simulink model "PMSM_FOC_demo"  (R2016a)
settings: Solver=ode3  StartTime=0.0  StopTime=0.4  FixedStep=ts  RelTol=1e-3
InitFcn:
  | para_init;
values from neighbouring files (symbols this model uses):
  J = 0.15    [para_init.m]
  MotOpMod = 2    [para_init.m]
  n_max = 6000    [para_init.m]
  nMotOpSpdMod = 1000*2*pi/60    (= 104.71975512)    [para_init.m]
  pp = 6    [para_init.m]
  r_dq = tan(theta_mtpa)    [para_init.m]
  ts_cc = 1/f_cc    (= 0.0001)    [para_init.m]
  U_bat = 200    [para_init.m]
undefined symbols (not defined in the file or in its folder): sigbuilder_block
undefined symbols (not defined in the file): f_cc, i_max, i_min, Kc_id, Kc_iq, Kc_n, Ki_id, Ki_iq, Ki_n, Kp_id, Kp_iq, Kp_n, Lamda_pm, lpa_cc, lpb_cc, Ls_d, Ls_q, rs, Te_max, Te_min, theta0, ts
libraries: simulink x2, simulink_extras x1
(part 1 of 2)
settings Model: Creator=Xinmei  LastModifiedBy=xinmei
settings DataIOCC: LimitDataPoints=on  SaveFormat=Array  SignalLoggingSaveFormat=ModelDataLogs
settings OptimizationCC: ExpressionDepthLimit=2147483647  EfficientMapNaN2IntZero=off
settings DebuggingCC: UnderspecifiedInitializationDetection=Classic  MergeDetectMultiDrivingBlocksExec=none  SolverPrmCheckMsg=warning  InheritedTsInSrcMsg=none  FcnCallInpInsideContextMsg=UseLocalSettings  StateNameClashWarn=warning
settings HardwareCC: ProdBitPerPointer=32  ProdLargestAtomicFloat=None  ProdIntDivRoundTo=Undefined  ProdEndianess=Unspecified  ProdWordSize=32  ProdHWDeviceType=32-bit Generic  TargetBitPerPointer=64  TargetLongLongMode=on  TargetIntDivRoundTo=Zero  TargetEndianess=LittleEndian  TargetWordSize=64  TargetHWDeviceType=MATLAB Host  ProdEqTarget=off
settings ModelReferenceCC: PropagateSignalLabelsOutOfModel=off
settings CodeAppCC: MaxIdLength=128
settings GRTTargetCC: CombineOutputUpdateFcns=off  GRTInterface=on
settings ConfigComp: CovModelRefEnable=Off

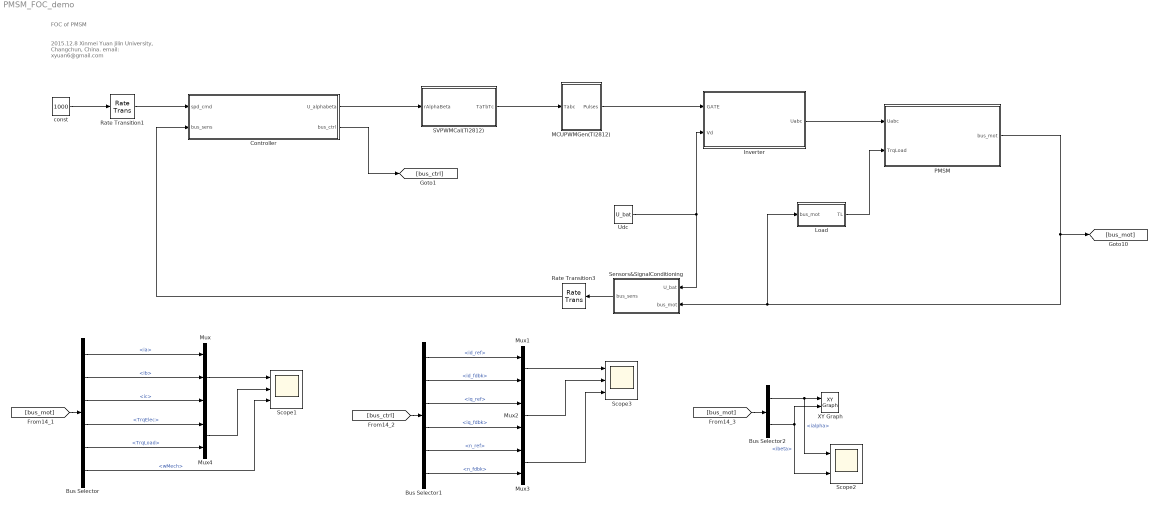
== system PMSM_FOC_demo ==
  note: 2015.12.8 Xinmei Yuan
      | Jilin University, Changchun, China.
      | email: xyuan6@gmail.com
  note: FOC of PMSM
  Bus Selector : BusSelector  OutputSignals=ia,ib,ic,TrqElec,TrqLoad,wMech
  Bus Selector1 : BusSelector  OutputSignals=id_ref,id_fdbk,iq_ref,iq_fdbk,n_ref,n_fdbk
  Bus Selector2 : BusSelector  OutputSignals=ialpha,ibeta
  Controller : Subsystem
  Inverter : Subsystem
      mask Display:
      | %image (imread('IGBT.jpg'))
      | port_label('input',1,'Gate'  )
      | port_label('input',2,'Udc'  )
      | port_label('output',1,'Uabc')
  Load : Subsystem
  MCUPWMGen(TI2812) : Subsystem  mask{fpwm=f_cc, nbit=16, Pulselim=0}
      mask prompts: fpwm "Chopping frequency(Hz)"; nbit "MCU PWM bits (ie: 16bits)"; Pulselim "PWM Pulse filtered"
  Mux : Mux  Inputs=3
  Mux{1..4} (4 alike) : Mux  Inputs=2
  PMSM : Subsystem  mask{r=rs, Ld=Ls_d, Lq=Ls_q, lamdaPM=Lamda_pm, J=J, p=pp, Thetam_init=theta0}
      mask prompts: r "Resistance (Ohm)"; Ld "Inductance Ld (H)"; Lq "Inductance Lq (H)"; lamdaPM "Flux induced by magnets (Wb)"; J "Inertia (kg*m^2)"; p "Pairs of poles"; Thetam_init "Rotor Initial Angle (rad)"
      mask Display:
      | %image (imread('Motor.jpg'))
      | port_label('input',1,'Uabc'  )
      | port_label('input',2,'T_L'  )
      | port_label('output',1,'bus_mot')
  Rate Transition1 : RateTransition  Integrity=off  OutPortSampleTime=ts_cc
  Rate Transition3 : RateTransition  Integrity=off  OutPortSampleTime=ts_cc
  SVPWMCal(TI2812) : Subsystem  mask{fpwm=f_cc}
      mask prompts: fpwm "Chopping frequency (Hz):"
      mask Display:
      | %image (imread('SVPWM.jpg'))
      | port_label('input',1,'rAlphaBeta'  )
      | port_label('output',1,'Tabc')
  Scope1 : Scope  NumInputPorts=3
  Scope2 : Scope  NumInputPorts=2
  Scope3 : Scope  NumInputPorts=3
  Sensors&SignalConditioning : Subsystem
  Udc : Constant  Value=U_bat  SampleTime=0
  XY Graph : simulink/Sinks/XY Graph  xmin=-150  xmax=150  ymin=-150  ymax=150  st=-1
  const : Constant  Value=1000  SampleTime=0
  wires:
  MCUPWMGen(TI2812)/1(Pulses) -> Inverter/1(GATE)
  Inverter/1(Uabc) -> PMSM/1(Uabc)
  SVPWMCal(TI2812)/1(TaTbTc) -> MCUPWMGen(TI2812)/1(Tabc)
  Udc/1 -> Sensors&SignalConditioning/1(U_bat), Inverter/2(Vd)
  PMSM/1(bus_mot) -> Load/1(bus_mot), Sensors&SignalConditioning/2(bus_mot), [bus_mot]
  [bus_mot] -> Bus Selector/1
  Bus Selector/3 -> Mux/3  "<ic>"
  Bus Selector/2 -> Mux/2  "<ib>"
  Bus Selector/1 -> Mux/1  "<ia>"
  Mux/1 -> Scope1/1
  Bus Selector/6 -> Scope1/3  "<wMech>"
  Load/1(TL) -> PMSM/2(TrqLoad)
  Sensors&SignalConditioning/1(bus_sens) -> Rate Transition3/1
  Rate Transition3/1 -> Controller/2(bus_sens)
  Controller/1(U_alphabeta) -> SVPWMCal(TI2812)/1(rAlphaBeta)
  const/1 -> Rate Transition1/1
  Rate Transition1/1 -> Controller/1(spd_cmd)
  [bus_ctrl] -> Bus Selector1/1
  Controller/2(bus_ctrl) -> [bus_ctrl]
  Bus Selector1/1 -> Mux1/1  "<id_ref>"
  Bus Selector1/2 -> Mux1/2  "<id_fdbk>"
  Bus Selector1/3 -> Mux2/1  "<iq_ref>"
  Bus Selector1/4 -> Mux2/2  "<iq_fdbk>"
  Mux1/1 -> Scope3/1
  Mux2/1 -> Scope3/2
  Bus Selector1/5 -> Mux3/1  "<n_ref>"
  Bus Selector1/6 -> Mux3/2  "<n_fdbk>"
  Mux3/1 -> Scope3/3
  Bus Selector/4 -> Mux4/1  "<TrqElec>"
  Bus Selector/5 -> Mux4/2  "<TrqLoad>"
  Mux4/1 -> Scope1/2
  [bus_mot] -> Bus Selector2/1
  Bus Selector2/1 -> Scope2/1, XY Graph/1  "<ialpha>"
  Bus Selector2/2 -> XY Graph/2, Scope2/2  "<ibeta>"

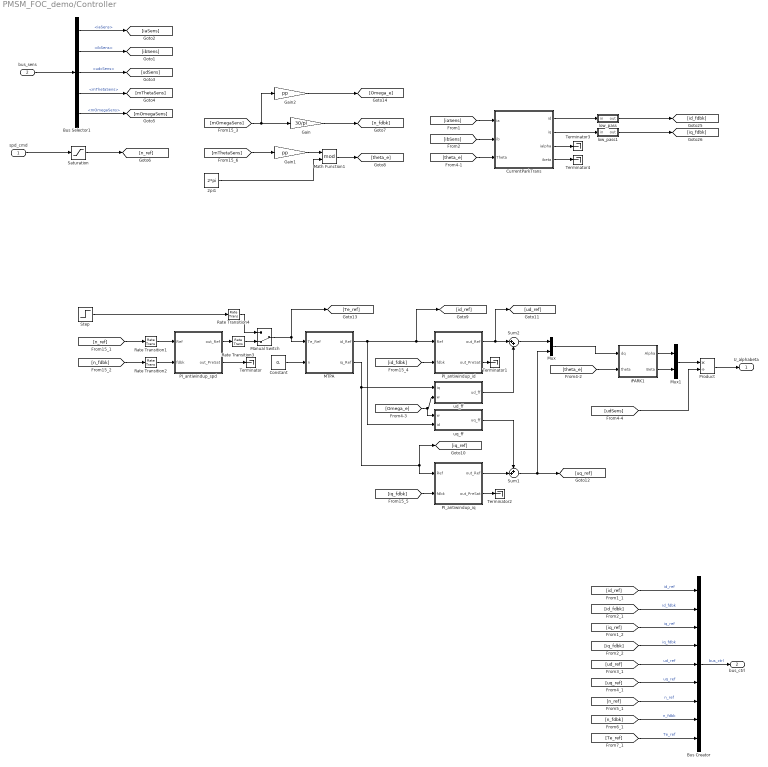
== system PMSM_FOC_demo/Controller ==
  spd_cmd : Inport
  bus_sens : Inport  Port=2
  2pi1 : Constant  Value=2*pi  SampleTime=ts_cc
  Bus Creator : BusCreator  Inputs=9
  Bus Selector1 : BusSelector  OutputSignals=iaSens,ibSens,udcSens,mThetaSens,mOmegaSens
  Constant : Constant  Value=0.  SampleTime=0
  CurrentParkTrans : Subsystem
  Gain : Gain  Gain=30/pi  SaturateOnIntegerOverflow=on  OutDataTypeStr=Inherit: Same as input  ParamDataTypeStr=Inherit: Same as input
  Gain1 : Gain  Gain=pp  SaturateOnIntegerOverflow=on  OutDataTypeStr=Inherit: Same as input  ParamDataTypeStr=Inherit: Same as input
  Gain2 : Gain  Gain=pp  SaturateOnIntegerOverflow=on  OutDataTypeStr=Inherit: Same as input  ParamDataTypeStr=Inherit: Same as input
  MTPA : Subsystem
  Manual Switch : ManualSwitch  CurrentSetting=0
  Math Function1 : Math  Operator=mod  SaturateOnIntegerOverflow=on
  Mux : Mux  Inputs=2
  Mux1 : Mux  Inputs=2
  PI_antiwindup_id : Subsystem  mask(PI Controller){P=Kp_id, I=Ki_id, sat=[i_min,i_max], Kc=Kc_id}
      mask prompts: P "Proportional:"; I "Integral"; sat "Minimum and maximum outputs:"
      mask init:
      | min=sat(1);max=sat(2);
  PI_antiwindup_iq : Subsystem  mask(PI Controller){P=Kp_iq, I=Ki_iq, sat=[i_min,i_max], Kc=Kc_iq}
      mask prompts: P "Proportional:"; I "Integral"; sat "Minimum and maximum outputs:"
      mask init:
      | min=sat(1);max=sat(2);
  PI_antiwindup_spd : Subsystem  mask(PI Controller){P=Kp_n, I=Ki_n, sat=[Te_min,Te_max], Kc=Kc_n}
      mask prompts: P "Proportional:"; I "Integral"; sat "Minimum and maximum outputs:"
      mask init:
      | min=sat(1);max=sat(2);
  Product : Product  Inputs=*/  SaturateOnIntegerOverflow=on  OutDataTypeStr=Inherit: Same as first input
  Rate Transition1 : RateTransition  Integrity=off  OutPortSampleTime=ts_sc
  Rate Transition2 : RateTransition  Integrity=off  OutPortSampleTime=ts_sc
  Rate Transition3 : RateTransition  Integrity=off  OutPortSampleTime=ts_cc
  Rate Transition4 : RateTransition  Integrity=off  OutPortSampleTime=ts_cc
  Saturation : Saturate  UpperLimit=n_max  LowerLimit=-n_max
  Step : Step  Time=0.5  After=10  SampleTime=ts_cc
  Sum1 : Sum  Inputs=++|
  Sum2 : Sum  Inputs=|++
  Terminator{,1..4} (5 alike) : Terminator
  iPARK1 : Subsystem
  low_pass : Subsystem  mask{a=lpa_cc, b=lpb_cc}
  low_pass1 : Subsystem  mask{a=lpa_cc, b=lpb_cc}
  ud_ff : Subsystem  mask{Lq=Ls_q}
  uq_ff : Subsystem  mask{Ld=Ls_d, lamdaPM=Lamda_pm}
  U_alphabeta : Outport
  bus_ctrl : Outport  Port=2
  wires:
  bus_sens/1 -> Bus Selector1/1
  Bus Selector1/1 -> [iaSens]  "<iaSens>"
  Bus Selector1/2 -> [ibSens]  "<ibSens>"
  Bus Selector1/3 -> [udSens]  "<udcSens>"
  Bus Selector1/4 -> [mThetaSens]  "<mThetaSens>"
  Bus Selector1/5 -> [mOmegaSens]  "<mOmegaSens>"
  [mOmegaSens] -> Gain2/1, Gain/1
  Gain/1 -> [n_fdbk]
  Saturation/1 -> [n_ref]
  [n_ref] -> Rate Transition1/1
  [n_fdbk] -> Rate Transition2/1
  PI_antiwindup_spd/2(out_PreSat) -> Terminator/1
  Constant/1 -> MTPA/2(n)
  Step/1 -> Rate Transition4/1
  PI_antiwindup_spd/1(out_Ref) -> Rate Transition3/1
  [id_fdbk] -> PI_antiwindup_id/2(fdbk)
  MTPA/1(id_Ref) -> uq_ff/2(id), [id_ref], PI_antiwindup_id/1(Ref)
  [iq_fdbk] -> PI_antiwindup_iq/2(fdbk)
  MTPA/2(iq_Ref) -> ud_ff/1(iq), PI_antiwindup_iq/1(Ref), [iq_ref]
  PI_antiwindup_id/2(out_PreSat) -> Terminator1/1
  PI_antiwindup_iq/2(out_PreSat) -> Terminator2/1
  Mux/1 -> iPARK1/1(dq)
  [theta_e] -> CurrentParkTrans/3(Theta)
  CurrentParkTrans/1(id) -> low_pass/1(in)
  CurrentParkTrans/2(iq) -> low_pass1/1(in)
  [iaSens] -> CurrentParkTrans/1(ia)
  [ibSens] -> CurrentParkTrans/2(ib)
  [mThetaSens] -> Gain1/1
  Gain1/1 -> Math Function1/1
  Math Function1/1 -> [theta_e]
  CurrentParkTrans/3(ialpha) -> Terminator3/1
  CurrentParkTrans/4(ibeta) -> Terminator4/1
  [theta_e] -> iPARK1/2(theta)
  2pi1/1 -> Math Function1/2
  Bus Creator/1 -> bus_ctrl/1  "bus_ctrl"
  [id_ref] -> Bus Creator/1  "id_ref"
  [id_fdbk] -> Bus Creator/2  "id_fdbk"
  [iq_ref] -> Bus Creator/3  "iq_ref"
  [iq_fdbk] -> Bus Creator/4  "iq_fdbk"
  Mux1/1 -> Product/1
  iPARK1/1(Alpha) -> Mux1/1
  iPARK1/2(Beta) -> Mux1/2
  [ud_ref] -> Bus Creator/5  "ud_ref"
  [uq_ref] -> Bus Creator/6  "uq_ref"
  low_pass/1(out) -> [id_fdbk]
  low_pass1/1(out) -> [iq_fdbk]
  [Omega_e] -> uq_ff/1(w), ud_ff/2(w)
  PI_antiwindup_id/1(out_Ref) -> Sum2/1, [ud_ref]
  uq_ff/1(uq_ff) -> Sum1/1
  PI_antiwindup_iq/1(out_Ref) -> Sum1/2
  ud_ff/1(ud_ff) -> Sum2/2
  Product/1 -> U_alphabeta/1
  [udSens] -> Product/2
  Sum2/1 -> Mux/1
  Sum1/1 -> Mux/2, [uq_ref]
  spd_cmd/1 -> Saturation/1
  Rate Transition2/1 -> PI_antiwindup_spd/2(fdbk)
  Manual Switch/1 -> MTPA/1(Te_Ref), [Te_ref]
  Rate Transition3/1 -> Manual Switch/2
  [n_ref] -> Bus Creator/7  "n_ref"
  [n_fdbk] -> Bus Creator/8  "n_fdbk"
  [Te_ref] -> Bus Creator/9  "Te_ref"
  Rate Transition1/1 -> PI_antiwindup_spd/1(Ref)
  Rate Transition4/1 -> Manual Switch/1
  Gain2/1 -> [Omega_e]

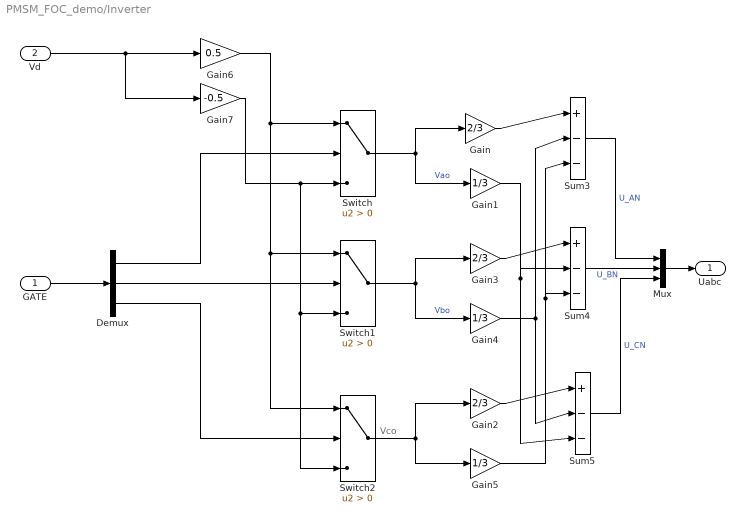
== system PMSM_FOC_demo/Inverter ==
  note: Vco
  GATE : Inport
  Vd : Inport  Port=2
  Demux : Demux  Outputs=3
  Gain : Gain  Gain=2/3  SaturateOnIntegerOverflow=on  OutDataTypeStr=Inherit: Same as input  ParamDataTypeStr=Inherit: Same as input
  Gain1 : Gain  Gain=1/3  SaturateOnIntegerOverflow=on  OutDataTypeStr=Inherit: Same as input  ParamDataTypeStr=Inherit: Same as input
  Gain2 : Gain  Gain=2/3  SaturateOnIntegerOverflow=on  OutDataTypeStr=Inherit: Same as input  ParamDataTypeStr=Inherit: Same as input
  Gain3 : Gain  Gain=2/3  SaturateOnIntegerOverflow=on  OutDataTypeStr=Inherit: Same as input  ParamDataTypeStr=Inherit: Same as input
  Gain4 : Gain  Gain=1/3  SaturateOnIntegerOverflow=on  OutDataTypeStr=Inherit: Same as input  ParamDataTypeStr=Inherit: Same as input
  Gain5 : Gain  Gain=1/3  SaturateOnIntegerOverflow=on  OutDataTypeStr=Inherit: Same as input  ParamDataTypeStr=Inherit: Same as input
  Gain6 : Gain  Gain=0.5  SaturateOnIntegerOverflow=on  OutDataTypeStr=Inherit: Same as input  ParamDataTypeStr=Inherit: Same as input
  Gain7 : Gain  Gain=-0.5  SaturateOnIntegerOverflow=on  OutDataTypeStr=Inherit: Same as input  ParamDataTypeStr=Inherit: Same as input
  Mux : Mux  Inputs=3
  Sum3 : Sum  Inputs=|+--  SaturateOnIntegerOverflow=on
  Sum4 : Sum  Inputs=|+--  SaturateOnIntegerOverflow=on
  Sum5 : Sum  Inputs=|+--  SaturateOnIntegerOverflow=on
  Switch : Switch  Criteria=u2 > Threshold  SaturateOnIntegerOverflow=on
  Switch1 : Switch  Criteria=u2 > Threshold  SaturateOnIntegerOverflow=on
  Switch2 : Switch  Criteria=u2 > Threshold  SaturateOnIntegerOverflow=on
  Uabc : Outport
  wires:
  GATE/1 -> Demux/1
  Demux/3 -> Switch2/2
  Demux/2 -> Switch1/2
  Demux/1 -> Switch/2
  Mux/1 -> Uabc/1
  Sum5/1 -> Mux/3  "U_CN"
  Sum4/1 -> Mux/2  "U_BN"
  Sum3/1 -> Mux/1  "U_AN"
  Vd/1 -> Gain7/1, Gain6/1
  Gain2/1 -> Sum5/1
  Gain1/1 -> Sum5/3, Sum4/2
  Gain3/1 -> Sum4/1
  Gain5/1 -> Sum4/3, Sum3/3
  Gain4/1 -> Sum5/2, Sum3/2
  Gain/1 -> Sum3/1
  Switch2/1 -> Gain5/1, Gain2/1
  Switch1/1 -> Gain4/1, Gain3/1  "Vbo"
  Switch/1 -> Gain1/1, Gain/1  "Vao"
  Gain7/1 -> Switch1/3, Switch2/3, Switch/3
  Gain6/1 -> Switch1/1, Switch2/1, Switch/1

== system PMSM_FOC_demo/Load ==
  bus_mot : Inport
  Bus Selector : BusSelector  OutputSignals=wMech
  Constant : Constant  Value=0  SampleTime=0
  Gain : Gain  Gain=30/pi  SaturateOnIntegerOverflow=on  OutDataTypeStr=Inherit: Same as input  ParamDataTypeStr=Inherit: Same as input
  Gain1 : Gain  Gain=0.01  SaturateOnIntegerOverflow=on  OutDataTypeStr=Inherit: Same as input  ParamDataTypeStr=Inherit: Same as input
  Manual Switch : ManualSwitch  CurrentSetting=0
  Signal Builder : Subsystem  Tag=STV Subsys  LoadFcn=sigbuilder_block('load');  StartFcn=sigbuilder_block('start');  StopFcn=sigbuilder_block('stop');  ClipboardFcn=sigbuilder_block('clipboard');  mask(Sigbuilder block){}
      mask help: Simulink:masks:SigbuilderBlock_MD
      mask init:
      | if ~strcmp(get_param(bdroot(gcbh),'SimulationStatus'),'stopped') tuvar = sigbuilder_block('maskInit'); end
      settings: CopyFcn=sigbuilder_block('copy');  DeleteFcn=sigbuilder_block('delete');  ModelCloseFcn=sigbuilder_block('modelClose');  PreSaveFcn=sigbuilder_block('preSave');  PauseFcn=sigbuilder_block('pause');  ContinueFcn=sigbuilder_block('continue');  NameChangeFcn=sigbuilder_block('namechange');  OpenFcn=sigbuilder_block('open',[437.25 199.5 550.5 399.75 ]);  CloseFcn=sigbuilder_block('close');
      mask Display: plot(0, 0, 100, 100,[2, 2, 32, 32, 2], [68, 8, 8, 68, 68],[32, 2], [38, 38], [32, 19, 2],[53, 60, 44], [32, 17, 17, 2],[16, 16, 31, 31]);txt = getActiveGroup(gcbh);text(2, 100, txt,'verticalAlignment', 'top');
  Sum : Sum  Inputs=|++
  TL : Outport
  wires:
  Bus Selector/1 -> [wMech]  "<wMech>"
  bus_mot/1 -> Bus Selector/1
  [wMech] -> Gain/1
  Gain/1 -> Gain1/1
  Gain1/1 -> Sum/1
  Sum/1 -> TL/1
  Constant/1 -> Manual Switch/1
  Manual Switch/1 -> Sum/2
  Signal Builder/1(Imported_Signal 1) -> Manual Switch/2

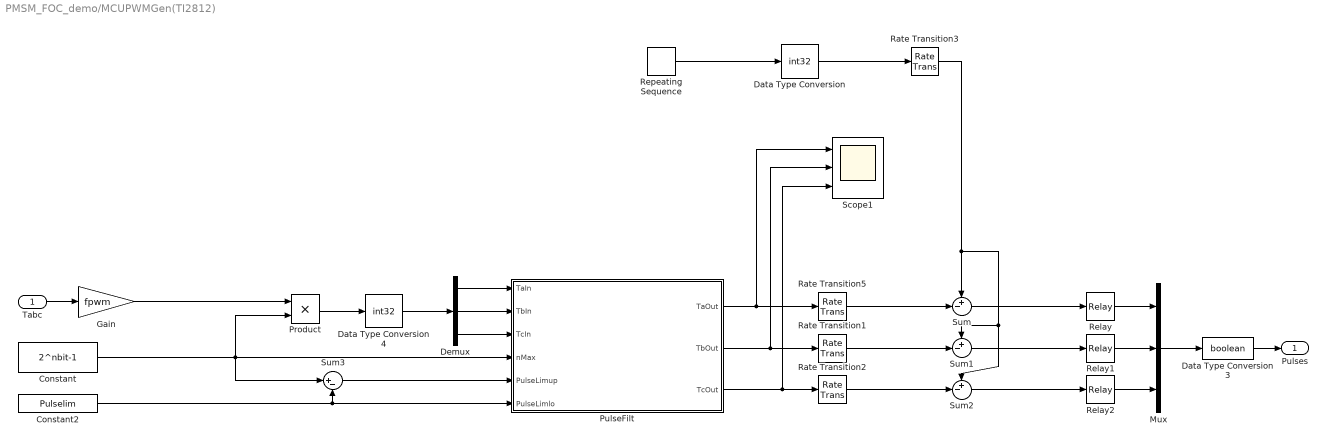
== system PMSM_FOC_demo/MCUPWMGen(TI2812) ==
  Tabc : Inport
  Constant : Constant  Value=2^nbit-1
  Constant2 : Constant  Value=Pulselim
  Data Type Conversion : DataTypeConversion  OutDataTypeStr=int32
  Data Type Conversion3 : DataTypeConversion  OutDataTypeStr=boolean
  Data Type Conversion4 : DataTypeConversion  OutDataTypeStr=int32
  Demux : Demux  Outputs=3
  Gain : Gain  Gain=fpwm
  Mux : Mux  Inputs=3
  Product : Product  RndMeth=Zero
  PulseFilt : Stateflow chart  TreatAsAtomicUnit=on
  Rate Transition{1..3,5} (4 alike) : RateTransition  Integrity=off  OutPortSampleTime=0
  Relay : Relay  OnSwitchValue=1  OffSwitchValue=-1
  Relay1 : Relay  OnSwitchValue=1  OffSwitchValue=-1
  Relay2 : Relay  OnSwitchValue=1  OffSwitchValue=-1
  Repeating Sequence : simulink/Sources/Repeating Sequence  rep_seq_t=[0 1/2/fpwm 1/fpwm]  rep_seq_y=[0 2^nbit-1 0]
  Scope1 : Scope  NumInputPorts=3
  Sum : Sum  Inputs=+-|
  Sum1 : Sum  Inputs=+-|
  Sum2 : Sum  Inputs=+-|
  Sum3 : Sum  Inputs=|+-
  Pulses : Outport
  wires:
  Data Type Conversion3/1 -> Pulses/1
  Repeating Sequence/1 -> Data Type Conversion/1
  Mux/1 -> Data Type Conversion3/1
  Tabc/1 -> Gain/1
  Relay2/1 -> Mux/3
  Relay1/1 -> Mux/2
  Relay/1 -> Mux/1
  Sum2/1 -> Relay2/1
  Sum1/1 -> Relay1/1
  Sum/1 -> Relay/1
  Data Type Conversion/1 -> Rate Transition3/1
  PulseFilt/1(TaOut) -> Scope1/1, Rate Transition5/1
  PulseFilt/2(TbOut) -> Scope1/2, Rate Transition1/1
  PulseFilt/3(TcOut) -> Scope1/3, Rate Transition2/1
  Data Type Conversion4/1 -> Demux/1
  Product/1 -> Data Type Conversion4/1
  Gain/1 -> Product/1
  Constant/1 -> Product/2, PulseFilt/4(nMax), Sum3/1
  Demux/1 -> PulseFilt/1(TaIn)
  Demux/2 -> PulseFilt/2(TbIn)
  Demux/3 -> PulseFilt/3(TcIn)
  Sum3/1 -> PulseFilt/5(PulseLimup)
  Constant2/1 -> PulseFilt/6(PulseLimlo), Sum3/2
  Rate Transition5/1 -> Sum/2
  Rate Transition1/1 -> Sum1/2
  Rate Transition2/1 -> Sum2/2
  Rate Transition3/1 -> Sum/1, Sum2/1, Sum1/1

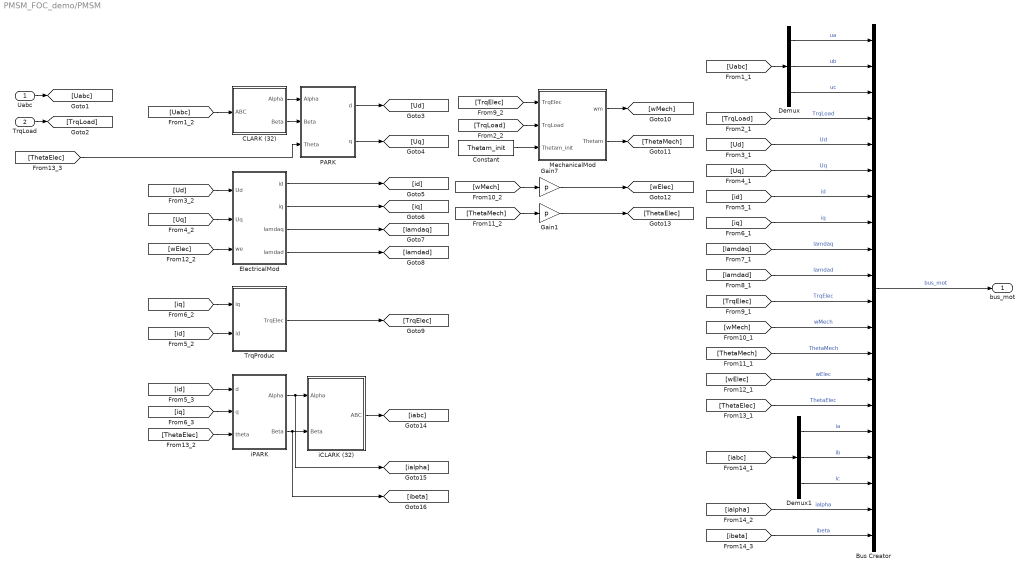
== system PMSM_FOC_demo/PMSM ==
  Uabc : Inport
  TrqLoad : Inport  Port=2
  Bus Creator : BusCreator  Inputs=20
  CLARK (32) : Subsystem
  Constant : Constant  Value=Thetam_init  SampleTime=[0, 0]
  Demux : Demux  Outputs=3
  Demux1 : Demux  Outputs=3
  ElectricalMod : Subsystem  mask{r=r, Ld=Ld, Lq=Lq, lamdaPM=lamdaPM}
      mask prompts: r "Stator resistance"; Ld "d axis inductance"; Lq "q axis inductance"; lamdaPM "Flux induced by magnets"
  Gain1 : Gain  Gain=p  SaturateOnIntegerOverflow=on  OutDataTypeStr=Inherit: Same as input  ParamDataTypeStr=Inherit: Same as input
  Gain7 : Gain  Gain=p  SaturateOnIntegerOverflow=on  OutDataTypeStr=Inherit: Same as input  ParamDataTypeStr=Inherit: Same as input
  MechanicalMod : Subsystem  mask{J=J}
      mask prompts: J "Intertia (kg*m^2)"
  PARK : Subsystem
  TrqProduc : Subsystem  mask{Ld=Ld, Lq=Lq, lamdaPM=lamdaPM, p=p}
      mask prompts: Ld "d Axis inductance"; Lq "q Axis inductance"; lamdaPM "Flux induced by magnets"; p "Pairs of poles"
  iCLARK (32) : Subsystem
  iPARK : Subsystem
  bus_mot : Outport
  wires:
  Bus Creator/1 -> bus_mot/1  "bus_mot"
  Demux1/3 -> Bus Creator/18  "ic"
  Demux1/2 -> Bus Creator/17  "ib"
  Demux1/1 -> Bus Creator/16  "ia"
  [ThetaElec] -> Bus Creator/15  "ThetaElec"
  [wElec] -> Bus Creator/14  "wElec"
  [ThetaMech] -> Bus Creator/13  "ThetaMech"
  [wMech] -> Bus Creator/12  "wMech"
  [TrqElec] -> Bus Creator/11  "TrqElec"
  [lamdad] -> Bus Creator/10  "lamdad"
  [lamdaq] -> Bus Creator/9  "lamdaq"
  [iq] -> Bus Creator/8  "iq"
  [id] -> Bus Creator/7  "id"
  [Uq] -> Bus Creator/6  "Uq"
  [Ud] -> Bus Creator/5  "Ud"
  [TrqLoad] -> Bus Creator/4  "TrqLoad"
  Demux/3 -> Bus Creator/3  "uc"
  Demux/2 -> Bus Creator/2  "ub"
  Demux/1 -> Bus Creator/1  "ua"
  [iabc] -> Demux1/1
  [Uabc] -> Demux/1
  [ThetaElec] -> iPARK/3(theta)
  [id] -> iPARK/1(d)
  iCLARK (32)/1(ABC) -> [iabc]
  [wElec] -> ElectricalMod/3(we)
  [ThetaMech] -> Gain1/1
  Gain7/1 -> [wElec]
  [wMech] -> Gain7/1
  MechanicalMod/2(Thetam) -> [ThetaMech]
  MechanicalMod/1(wm) -> [wMech]
  ElectricalMod/4(lamdad) -> [lamdad]
  ElectricalMod/3(lamdaq) -> [lamdaq]
  Constant/1 -> MechanicalMod/3(Thetam_init)
  [TrqLoad] -> MechanicalMod/2(TrqLoad)
  [TrqElec] -> MechanicalMod/1(TrqElec)
  TrqProduc/1(TrqElec) -> [TrqElec]
  ElectricalMod/2(iq) -> [iq]
  ElectricalMod/1(id) -> [id]
  [Uq] -> ElectricalMod/2(Uq)
  [Ud] -> ElectricalMod/1(Ud)
  PARK/2(q) -> [Uq]
  PARK/1(d) -> [Ud]
  TrqLoad/1 -> [TrqLoad]
  [Uabc] -> CLARK (32)/1(ABC)
  Uabc/1 -> [Uabc]
  [iq] -> TrqProduc/1(iq)
  [id] -> TrqProduc/2(id)
  CLARK (32)/1(Alpha) -> PARK/1(Alpha)
  CLARK (32)/2(Beta) -> PARK/2(Beta)
  [iq] -> iPARK/2(q)
  iPARK/1(Alpha) -> iCLARK (32)/1(Alpha), [ialpha]
  iPARK/2(Beta) -> iCLARK (32)/2(Beta), [ibeta]
  Gain1/1 -> [ThetaElec]
  [ThetaElec] -> PARK/3(Theta)
  [ialpha] -> Bus Creator/19  "ialpha"
  [ibeta] -> Bus Creator/20  "ibeta"

== system PMSM_FOC_demo/SVPWMCal(TI2812) ==
  note: Xinmei modified at June 2006
  note: Hoang Le-Huy
      | Universite Laval
      | Quebec
  note: Pierre Giroux, Gilbert Sybille
      | Power System Laboratory, IREQ
      | Hydro-Quebec
  note: Space Vector Pulse Width Modulation (SV PWM)
  rAlphaBeta : Inport
  Demux2 : Demux  Outputs=2
  INFO : Subsystem
      mask Display: disp('?')
  Subsystem : Subsystem
  TaTbTcCal : Subsystem
  sector : Subsystem
  t1 t2 : Subsystem
  ton : Subsystem
  TaTbTc : Outport
  wires:
  TaTbTcCal/1(TaTbTc) -> TaTbTc/1
  sector/1(sector) -> t1 t2/1(sector), TaTbTcCal/1(sector)
  Demux2/2 -> Subsystem/2(beta), sector/2(beta)
  Demux2/1 -> sector/1(afa), Subsystem/1(afa)
  Subsystem/1(XYZ) -> t1 t2/2(XYZ)
  ton/1(ton) -> TaTbTcCal/2(ton)
  t1 t2/1(t1 t2) -> ton/1(t1 t2)
  rAlphaBeta/1 -> Demux2/1

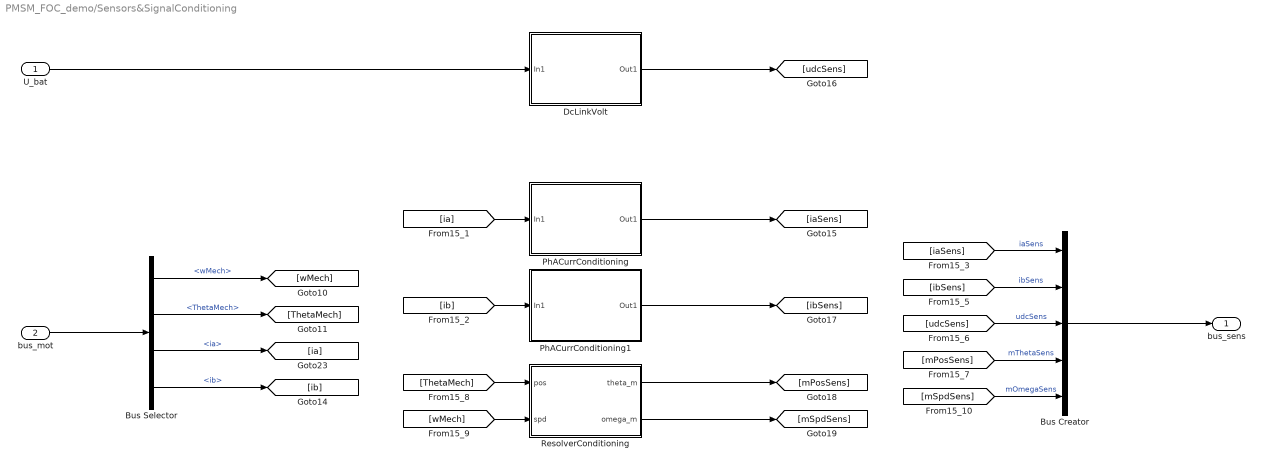
== system PMSM_FOC_demo/Sensors&SignalConditioning ==
  U_bat : Inport
  bus_mot : Inport  Port=2
  Bus Creator : BusCreator  Inputs=5
  Bus Selector : BusSelector  OutputSignals=wMech,ThetaMech,ia,ib
  DcLinkVolt : Subsystem  mask{Gain=1, Offset=0}
      mask Display:
      | %image (imread('VoltageSens.jpg'))
      | port_label('input',1,'ADin'  )
      | port_label('output',1,'Voltage')
  PhACurrConditioning : Subsystem  mask{Gain=1, Offset=0, bw=2000, Ts=ts}
      mask prompts: bw "Filter Bandwidth"; Ts "Filter Sample time"
      mask Display:
      | %image (imread('CurrentSens.jpg'))
      | port_label('input',1,'ADin'  )
      | port_label('output',1,'Current')
  PhACurrConditioning1 : Subsystem  mask{Gain=1, Offset=0, bw=2000, Ts=ts}
      mask prompts: bw "Filter Bandwidth"; Ts "Filter Sample time"
      mask Display:
      | %image (imread('CurrentSens.jpg'))
      | port_label('input',1,'ADin'  )
      | port_label('output',1,'Current')
  ResolverConditioning : Subsystem
      mask Display:
      | %image (imread('Resolver.jpg'))
      | %port_label('input',1,'sin'  )
      | %port_label('input',2,'cos'  )
      | %port_label('output',1,'Pos')
      | %port_label('output',2,'Spd')
      | 
      | port_label('input',1,'pos'  )
      | port_label('input',2,'spd'  )
      | port_label('output',1,'theta_m')
      | port_label('output',2,'omega_m')
  bus_sens : Outport
  wires:
  DcLinkVolt/1(Out1) -> [udcSens]
  Bus Selector/1 -> [wMech]  "<wMech>"
  Bus Selector/2 -> [ThetaMech]  "<ThetaMech>"
  Bus Selector/3 -> [ia]  "<ia>"
  Bus Selector/4 -> [ib]  "<ib>"
  bus_mot/1 -> Bus Selector/1
  PhACurrConditioning/1(Out1) -> [iaSens]
  PhACurrConditioning1/1(Out1) -> [ibSens]
  ResolverConditioning/1(theta_m) -> [mPosSens]
  [ia] -> PhACurrConditioning/1(In1)
  [ib] -> PhACurrConditioning1/1(In1)
  U_bat/1 -> DcLinkVolt/1(In1)
  [ThetaMech] -> ResolverConditioning/1(pos)
  [wMech] -> ResolverConditioning/2(spd)
  Bus Creator/1 -> bus_sens/1
  ResolverConditioning/2(omega_m) -> [mSpdSens]
  [iaSens] -> Bus Creator/1  "iaSens"
  [ibSens] -> Bus Creator/2  "ibSens"
  [mPosSens] -> Bus Creator/4  "mThetaSens"
  [udcSens] -> Bus Creator/3  "udcSens"
  [mSpdSens] -> Bus Creator/5  "mOmegaSens"

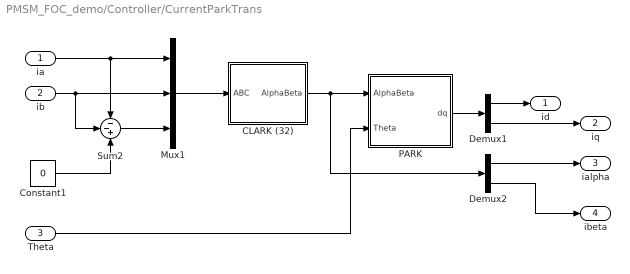
== system PMSM_FOC_demo/Controller/CurrentParkTrans ==
  ia : Inport
  ib : Inport  Port=2
  Theta : Inport  Port=3
  CLARK (32) : Subsystem
  Constant1 : Constant  Value=0  SampleTime=ts_cc
  Demux1 : Demux  Outputs=2
  Demux2 : Demux  Outputs=2
  Mux1 : Mux  Inputs=3
  PARK : Subsystem
  Sum2 : Sum  Inputs=--+
  id : Outport
  iq : Outport  Port=2
  ialpha : Outport  Port=3
  ibeta : Outport  Port=4
  wires:
  ia/1 -> Mux1/1, Sum2/1
  ib/1 -> Mux1/2, Sum2/2
  Constant1/1 -> Sum2/3
  Sum2/1 -> Mux1/3
  Mux1/1 -> CLARK (32)/1(ABC)
  CLARK (32)/1(AlphaBeta) -> PARK/1(AlphaBeta), Demux2/1
  PARK/1(dq) -> Demux1/1
  Demux1/1 -> id/1
  Demux1/2 -> iq/1
  Theta/1 -> PARK/2(Theta)
  Demux2/1 -> ialpha/1
  Demux2/2 -> ibeta/1

== system PMSM_FOC_demo/Controller/MTPA ==
  Te_Ref : Inport
  n : Inport  Port=2
  Te2Iq : Gain  Gain=1/0.68  SaturateOnIntegerOverflow=on  OutDataTypeStr=Inherit: Same as input  ParamDataTypeStr=Inherit: Same as input
  Te2Iq1 : Gain  Gain=-r_dq  SaturateOnIntegerOverflow=on  OutDataTypeStr=Inherit: Same as input  ParamDataTypeStr=Inherit: Same as input
  Terminator : Terminator
  id_Ref : Outport  InitialOutput=0
  iq_Ref : Outport  Port=2  InitialOutput=0
  wires:
  Te_Ref/1 -> Te2Iq/1
  Te2Iq/1 -> Te2Iq1/1, iq_Ref/1
  Te2Iq1/1 -> id_Ref/1
  n/1 -> Terminator/1

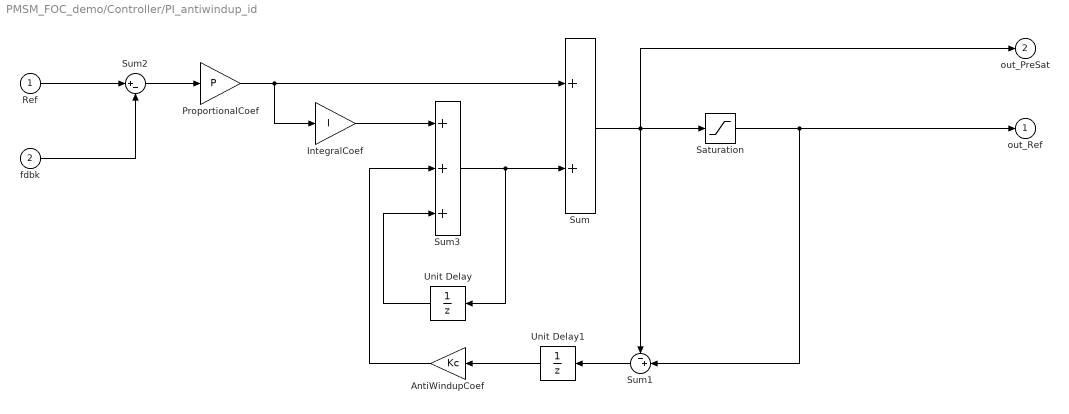
== system PMSM_FOC_demo/Controller/PI_antiwindup_id ==
  Ref : Inport
  fdbk : Inport  Port=2
  AntiWindupCoef : Gain  Gain=Kc  SaturateOnIntegerOverflow=on  OutDataTypeStr=Inherit: Same as input  ParamDataTypeStr=Inherit: Same as input
  IntegralCoef : Gain  Gain=I  SaturateOnIntegerOverflow=on  OutDataTypeStr=Inherit: Same as input  ParamDataTypeStr=Inherit: Same as input
  ProportionalCoef : Gain  Gain=P  SaturateOnIntegerOverflow=on  OutDataTypeStr=Inherit: Same as input  ParamDataTypeStr=Inherit: Same as input
  Saturation : Saturate  UpperLimit=max  LowerLimit=min
  Sum : Sum  SaturateOnIntegerOverflow=on  InputSameDT=on  OutDataTypeStr=Inherit: Same as first input
  Sum1 : Sum  Inputs=-+|
  Sum2 : Sum  Inputs=|+-
  Sum3 : Sum  Inputs=+++  SaturateOnIntegerOverflow=on  InputSameDT=on  OutDataTypeStr=Inherit: Same as first input
  Unit Delay : UnitDelay  SampleTime=-1
  Unit Delay1 : UnitDelay  SampleTime=-1
  out_Ref : Outport  InitialOutput=0
  out_PreSat : Outport  Port=2  InitialOutput=0
  wires:
  AntiWindupCoef/1 -> Sum3/2
  Unit Delay/1 -> Sum3/3
  Sum3/1 -> Sum/2, Unit Delay/1
  IntegralCoef/1 -> Sum3/1
  ProportionalCoef/1 -> IntegralCoef/1, Sum/1
  Saturation/1 -> Sum1/2, out_Ref/1
  Sum2/1 -> ProportionalCoef/1
  fdbk/1 -> Sum2/2
  Ref/1 -> Sum2/1
  Sum/1 -> out_PreSat/1, Sum1/1, Saturation/1
  Sum1/1 -> Unit Delay1/1
  Unit Delay1/1 -> AntiWindupCoef/1

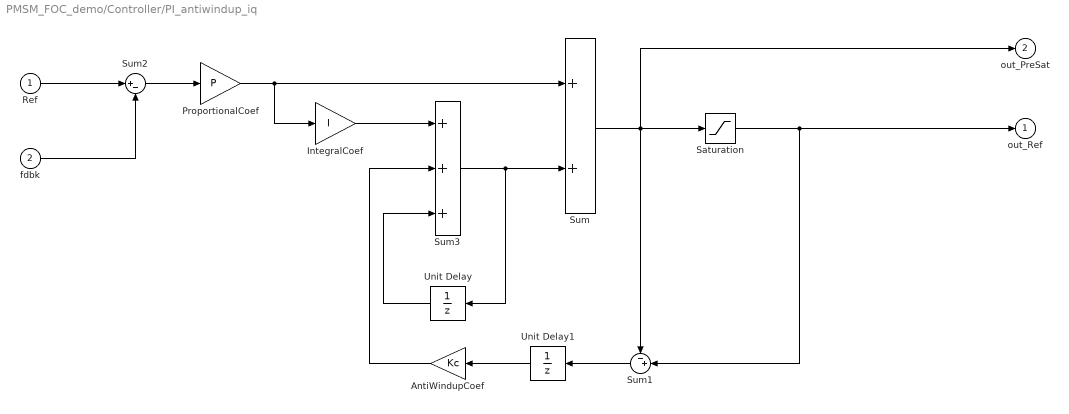
== system PMSM_FOC_demo/Controller/PI_antiwindup_iq ==
  Ref : Inport
  fdbk : Inport  Port=2
  AntiWindupCoef : Gain  Gain=Kc  SaturateOnIntegerOverflow=on  OutDataTypeStr=Inherit: Same as input  ParamDataTypeStr=Inherit: Same as input
  IntegralCoef : Gain  Gain=I  SaturateOnIntegerOverflow=on  OutDataTypeStr=Inherit: Same as input  ParamDataTypeStr=Inherit: Same as input
  ProportionalCoef : Gain  Gain=P  SaturateOnIntegerOverflow=on  OutDataTypeStr=Inherit: Same as input  ParamDataTypeStr=Inherit: Same as input
  Saturation : Saturate  UpperLimit=max  LowerLimit=min
  Sum : Sum  SaturateOnIntegerOverflow=on  InputSameDT=on  OutDataTypeStr=Inherit: Same as first input
  Sum1 : Sum  Inputs=-+|
  Sum2 : Sum  Inputs=|+-
  Sum3 : Sum  Inputs=+++  SaturateOnIntegerOverflow=on  InputSameDT=on  OutDataTypeStr=Inherit: Same as first input
  Unit Delay : UnitDelay  SampleTime=-1
  Unit Delay1 : UnitDelay  SampleTime=-1
  out_Ref : Outport  InitialOutput=0
  out_PreSat : Outport  Port=2  InitialOutput=0
  wires:
  Sum1/1 -> Unit Delay1/1
  Sum/1 -> Saturation/1, Sum1/1, out_PreSat/1
  Ref/1 -> Sum2/1
  fdbk/1 -> Sum2/2
  Sum2/1 -> ProportionalCoef/1
  Saturation/1 -> out_Ref/1, Sum1/2
  ProportionalCoef/1 -> Sum/1, IntegralCoef/1
  IntegralCoef/1 -> Sum3/1
  Sum3/1 -> Unit Delay/1, Sum/2
  Unit Delay/1 -> Sum3/3
  AntiWindupCoef/1 -> Sum3/2
  Unit Delay1/1 -> AntiWindupCoef/1

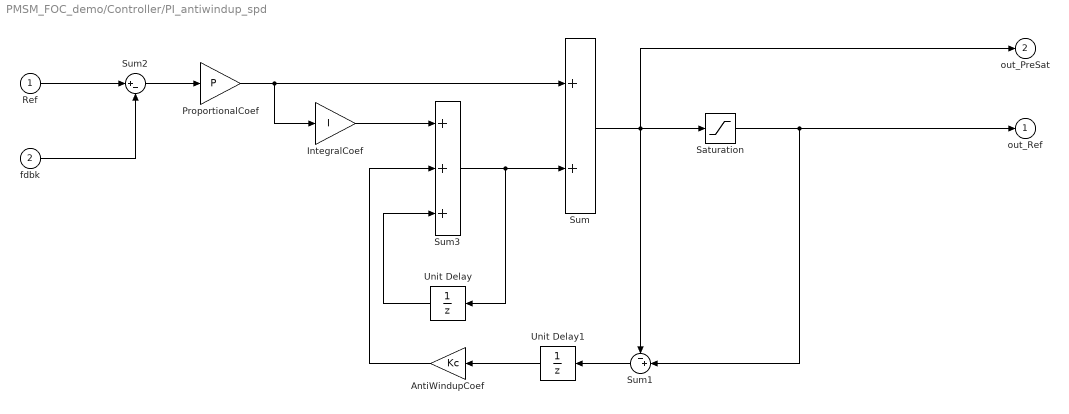
== system PMSM_FOC_demo/Controller/PI_antiwindup_spd ==
  Ref : Inport
  fdbk : Inport  Port=2
  AntiWindupCoef : Gain  Gain=Kc  SaturateOnIntegerOverflow=on  OutDataTypeStr=Inherit: Same as input  ParamDataTypeStr=Inherit: Same as input
  IntegralCoef : Gain  Gain=I  SaturateOnIntegerOverflow=on  OutDataTypeStr=Inherit: Same as input  ParamDataTypeStr=Inherit: Same as input
  ProportionalCoef : Gain  Gain=P  SaturateOnIntegerOverflow=on  OutDataTypeStr=Inherit: Same as input  ParamDataTypeStr=Inherit: Same as input
  Saturation : Saturate  UpperLimit=max  LowerLimit=min
  Sum : Sum  SaturateOnIntegerOverflow=on  InputSameDT=on  OutDataTypeStr=Inherit: Same as first input
  Sum1 : Sum  Inputs=-+|
  Sum2 : Sum  Inputs=|+-
  Sum3 : Sum  Inputs=+++  SaturateOnIntegerOverflow=on  InputSameDT=on  OutDataTypeStr=Inherit: Same as first input
  Unit Delay : UnitDelay  SampleTime=-1
  Unit Delay1 : UnitDelay  SampleTime=-1
  out_Ref : Outport  InitialOutput=0
  out_PreSat : Outport  Port=2  InitialOutput=0
  wires:
  Sum1/1 -> Unit Delay1/1
  Sum/1 -> Saturation/1, Sum1/1, out_PreSat/1
  Ref/1 -> Sum2/1
  fdbk/1 -> Sum2/2
  Sum2/1 -> ProportionalCoef/1
  Saturation/1 -> out_Ref/1, Sum1/2
  ProportionalCoef/1 -> Sum/1, IntegralCoef/1
  IntegralCoef/1 -> Sum3/1
  Sum3/1 -> Unit Delay/1, Sum/2
  Unit Delay/1 -> Sum3/3
  AntiWindupCoef/1 -> Sum3/2
  Unit Delay1/1 -> AntiWindupCoef/1

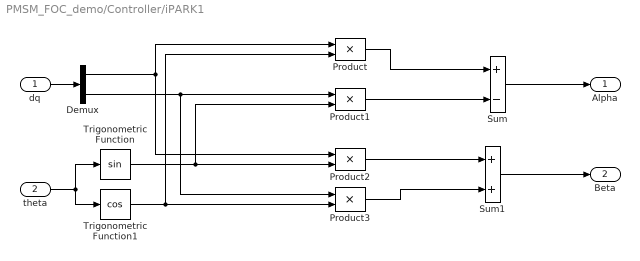
== system PMSM_FOC_demo/Controller/iPARK1 ==
  dq : Inport
  theta : Inport  Port=2
  Demux : Demux  Outputs=2
  Product{,1..3} (4 alike) : Product  SaturateOnIntegerOverflow=on  OutDataTypeStr=Inherit: Same as first input
  Sum : Sum  Inputs=+-  SaturateOnIntegerOverflow=on
  Sum1 : Sum  SaturateOnIntegerOverflow=on
  Trigonometric Function : Trigonometry
  Trigonometric Function1 : Trigonometry  Operator=cos
  Alpha : Outport
  Beta : Outport  Port=2
  wires:
  dq/1 -> Demux/1
  Demux/1 -> Product2/1, Product/1
  Demux/2 -> Product3/1, Product1/1
  Sum/1 -> Alpha/1
  Trigonometric Function/1 -> Product2/2, Product1/2
  Trigonometric Function1/1 -> Product3/2, Product/2
  theta/1 -> Trigonometric Function1/1, Trigonometric Function/1
  Product/1 -> Sum/1
  Product1/1 -> Sum/2
  Sum1/1 -> Beta/1
  Product2/1 -> Sum1/1
  Product3/1 -> Sum1/2

== system PMSM_FOC_demo/Controller/low_pass ==
  in : Inport
  Gain : Gain  Gain=a  SaturateOnIntegerOverflow=on  OutDataTypeStr=Inherit: Same as input  ParamDataTypeStr=Inherit: Same as input
  Gain1 : Gain  Gain=b  SaturateOnIntegerOverflow=on  OutDataTypeStr=Inherit: Same as input  ParamDataTypeStr=Inherit: Same as input
  Sum : Sum  Inputs=|++
  Sum1 : Sum  Inputs=|++
  Unit Delay : UnitDelay  SampleTime=-1
  Unit Delay1 : UnitDelay  SampleTime=-1
  out : Outport
  wires:
  Unit Delay/1 -> Gain/1
  in/1 -> Unit Delay1/1, Sum/1
  Unit Delay1/1 -> Sum/2
  Sum/1 -> Gain1/1
  Gain1/1 -> Sum1/1
  Gain/1 -> Sum1/2
  Sum1/1 -> Unit Delay/1, out/1

== system PMSM_FOC_demo/Controller/low_pass1 ==
  in : Inport
  Gain : Gain  Gain=a  SaturateOnIntegerOverflow=on  OutDataTypeStr=Inherit: Same as input  ParamDataTypeStr=Inherit: Same as input
  Gain1 : Gain  Gain=b  SaturateOnIntegerOverflow=on  OutDataTypeStr=Inherit: Same as input  ParamDataTypeStr=Inherit: Same as input
  Sum : Sum  Inputs=|++
  Sum1 : Sum  Inputs=|++
  Unit Delay : UnitDelay  SampleTime=-1
  Unit Delay1 : UnitDelay  SampleTime=-1
  out : Outport
  wires:
  Sum1/1 -> out/1, Unit Delay/1
  Gain/1 -> Sum1/2
  Gain1/1 -> Sum1/1
  Sum/1 -> Gain1/1
  Unit Delay1/1 -> Sum/2
  in/1 -> Sum/1, Unit Delay1/1
  Unit Delay/1 -> Gain/1

== system PMSM_FOC_demo/Controller/ud_ff ==
  iq : Inport
  w : Inport  Port=2
  Gain1 : Gain  Gain=Lq  SaturateOnIntegerOverflow=on  OutDataTypeStr=Inherit: Same as input  ParamDataTypeStr=Inherit: Same as input
  Gain2 : Gain  Gain=-1  SaturateOnIntegerOverflow=on  OutDataTypeStr=Inherit: Same as input  ParamDataTypeStr=Inherit: Same as input
  Product : Product  SaturateOnIntegerOverflow=on  OutDataTypeStr=Inherit: Same as first input
  ud_ff : Outport
  wires:
  Product/1 -> Gain2/1
  w/1 -> Product/1
  Gain1/1 -> Product/2
  iq/1 -> Gain1/1
  Gain2/1 -> ud_ff/1

== system PMSM_FOC_demo/Controller/uq_ff ==
  w : Inport
  id : Inport  Port=2
  Add : Sum
  Constant : Constant  Value=lamdaPM  SampleTime=0
  Gain1 : Gain  Gain=Ld  SaturateOnIntegerOverflow=on  OutDataTypeStr=Inherit: Same as input  ParamDataTypeStr=Inherit: Same as input
  Product : Product  SaturateOnIntegerOverflow=on  OutDataTypeStr=Inherit: Same as first input
  Rate Transition3 : RateTransition  Integrity=off  OutPortSampleTime=ts_cc
  uq_ff : Outport
  wires:
  Constant/1 -> Rate Transition3/1
  Add/1 -> Product/2
  Gain1/1 -> Add/1
  Product/1 -> uq_ff/1
  w/1 -> Product/1
  id/1 -> Gain1/1
  Rate Transition3/1 -> Add/2

== system PMSM_FOC_demo/Load/Signal Builder ==
  Demux : Demux  Tag=STV Demux  Outputs=1
  FromWs : FromWorkspace  Tag=STV FromWs  VariableName=tuvar  SampleTime=0
      SigBuilderData=|
      | common.afterFinalStr = 'Extrapolate'
      | common.sampleTime = 0
      | dataSet.timeRange = [0 19]
      | dataSet.name = 'Sheet1'
      | sbobj.Name = 'Signal Builder'
      | sbobj.Groups.Name = 'Sheet1'
      | sbobj.Groups.Signals.Name = 'Imported_Signal 1'
      | sbobj.Groups.Signals.XData = [0 3 3 5 5 7 7 9 9 11 11 13 13 15 15 17 17 19]
      | sbobj.Groups.Signals.YData = [0 0 6 6 0 0 12 12 0 0 18 18 0 0 24 24 0 0]
      | sbobj.Groups.TimeRange = [0 19]
  Imported_Signal 1 : Outport
  wires:
  Demux/1 -> Imported_Signal 1/1
  FromWs/1 -> Demux/1

== system PMSM_FOC_demo/PMSM/CLARK (32) ==
  ABC : Inport
  Demux : Demux  Outputs=3
  Gain : Gain  SaturateOnIntegerOverflow=on  OutDataTypeStr=Inherit: Same as input  ParamDataTypeStr=Inherit: Same as input
  Gain1 : Gain  Gain=1/2  SaturateOnIntegerOverflow=on  OutDataTypeStr=Inherit: Same as input  ParamDataTypeStr=Inherit: Same as input
  Gain2 : Gain  Gain=1/2  SaturateOnIntegerOverflow=on  OutDataTypeStr=Inherit: Same as input  ParamDataTypeStr=Inherit: Same as input
  Gain3 : Gain  Gain=sqrt(3)/2  SaturateOnIntegerOverflow=on  OutDataTypeStr=Inherit: Same as input  ParamDataTypeStr=Inherit: Same as input
  Gain4 : Gain  Gain=sqrt(3)/2  SaturateOnIntegerOverflow=on  OutDataTypeStr=Inherit: Same as input  ParamDataTypeStr=Inherit: Same as input
  Gain5 : Gain  Gain=2/3  SaturateOnIntegerOverflow=on  OutDataTypeStr=Inherit: Same as input  ParamDataTypeStr=Inherit: Same as input
  Sum : Sum  Inputs=+--  SaturateOnIntegerOverflow=on
  Sum1 : Sum  Inputs=+-  SaturateOnIntegerOverflow=on
  Alpha : Outport
  Beta : Outport  Port=2
  wires:
  Gain4/1 -> Sum1/2
  Gain3/1 -> Sum1/1
  Gain2/1 -> Sum/3
  Gain1/1 -> Sum/2
  Gain/1 -> Sum/1
  Demux/3 -> Gain4/1, Gain2/1
  Demux/2 -> Gain3/1, Gain1/1
  Demux/1 -> Gain/1
  ABC/1 -> Gain5/1
  Gain5/1 -> Demux/1
  Sum/1 -> Alpha/1
  Sum1/1 -> Beta/1

== system PMSM_FOC_demo/PMSM/ElectricalMod ==
  Ud : Inport
  Uq : Inport  Port=2
  we : Inport  Port=3
  dAxisVolEqu : Subsystem
  qAxisVolEqu : Subsystem
  id : Outport
  iq : Outport  Port=2
  lamdaq : Outport  Port=3
  lamdad : Outport  Port=4
  wires:
  qAxisVolEqu/2(lamdad) -> lamdad/1
  dAxisVolEqu/1(lamdaq) -> lamdaq/1
  Uq/1 -> qAxisVolEqu/3(Uq)
  qAxisVolEqu/1(iq) -> dAxisVolEqu/3(iq), iq/1
  dAxisVolEqu/2(id) -> qAxisVolEqu/1(id), id/1
  Ud/1 -> dAxisVolEqu/1(Ud)
  we/1 -> qAxisVolEqu/2(w), dAxisVolEqu/2(w)

== system PMSM_FOC_demo/PMSM/MechanicalMod ==
  TrqElec : Inport
  TrqLoad : Inport  Port=2
  Thetam_init : Inport  Port=3
  Constant : Constant  Value=MotOpMod  SampleTime=[0, 0]
  Constant1 : Constant  Value=nMotOpSpdMod  SampleTime=[0, 0]
  Gain7 : Gain  Gain=1/J  SaturateOnIntegerOverflow=on  OutDataTypeStr=Inherit: Same as input  ParamDataTypeStr=Inherit: Same as input
  Integrator : Integrator
  Integrator2 : Integrator  InitialConditionSource=external
  Multiport Switch : MultiPortSwitch  Inputs=2
  Sum1 : Sum  Inputs=+-  SaturateOnIntegerOverflow=on
  wm : Outport
  Thetam : Outport  Port=2
  wires:
  TrqElec/1 -> Sum1/1
  Thetam_init/1 -> Integrator2/2
  Integrator2/1 -> Thetam/1
  TrqLoad/1 -> Sum1/2
  Integrator/1 -> Multiport Switch/3
  Constant/1 -> Multiport Switch/1
  Multiport Switch/1 -> Integrator2/1, wm/1
  Constant1/1 -> Multiport Switch/2
  Sum1/1 -> Gain7/1
  Gain7/1 -> Integrator/1

== system PMSM_FOC_demo/PMSM/PARK ==
  Alpha : Inport
  Beta : Inport  Port=2
  Theta : Inport  Port=3
  Product{,1..3} (4 alike) : Product  SaturateOnIntegerOverflow=on  OutDataTypeStr=Inherit: Same as first input
  Sum : Sum  SaturateOnIntegerOverflow=on
  Sum1 : Sum  Inputs=-+  SaturateOnIntegerOverflow=on
  Trigonometric Function : Trigonometry  Operator=cos
  Trigonometric Function1 : Trigonometry
  d : Outport
  q : Outport  Port=2
  wires:
  Product3/1 -> Sum1/2
  Product1/1 -> Sum/2
  Beta/1 -> Product3/2, Product1/1
  Trigonometric Function1/1 -> Product2/2, Product1/2
  Product/1 -> Sum/1
  Trigonometric Function/1 -> Product3/1, Product/2
  Alpha/1 -> Product2/1, Product/1
  Sum1/1 -> q/1
  Theta/1 -> Trigonometric Function1/1, Trigonometric Function/1
  Sum/1 -> d/1
  Product2/1 -> Sum1/1

== system PMSM_FOC_demo/PMSM/TrqProduc ==
  iq : Inport
  id : Inport  Port=2
  Gain : Gain  Gain=p  SaturateOnIntegerOverflow=on  OutDataTypeStr=Inherit: Same as input  ParamDataTypeStr=Inherit: Same as input
  Gain1 : Gain  Gain=3/2  SaturateOnIntegerOverflow=on  OutDataTypeStr=Inherit: Same as input  ParamDataTypeStr=Inherit: Same as input
  Gain2 : Gain  Gain=lamdaPM  SaturateOnIntegerOverflow=on  OutDataTypeStr=Inherit: Same as input  ParamDataTypeStr=Inherit: Same as input
  Gain3 : Gain  Gain=Ld-Lq  SaturateOnIntegerOverflow=on  OutDataTypeStr=Inherit: Same as input  ParamDataTypeStr=Inherit: Same as input
  Product : Product  SaturateOnIntegerOverflow=on  OutDataTypeStr=Inherit: Same as first input
  Sum : Sum  SaturateOnIntegerOverflow=on
  TrqElec : Outport
  wires:
  Gain/1 -> Gain1/1
  Gain3/1 -> Sum/2
  Product/1 -> Gain3/1
  Gain2/1 -> Sum/1
  iq/1 -> Product/1, Gain2/1
  Sum/1 -> Gain/1
  id/1 -> Product/2
  Gain1/1 -> TrqElec/1

== system PMSM_FOC_demo/PMSM/iCLARK (32) ==
  Alpha : Inport
  Beta : Inport  Port=2
  Gain : Gain  SaturateOnIntegerOverflow=on  OutDataTypeStr=Inherit: Same as input  ParamDataTypeStr=Inherit: Same as input
  Gain1 : Gain  Gain=1/2  SaturateOnIntegerOverflow=on  OutDataTypeStr=Inherit: Same as input  ParamDataTypeStr=Inherit: Same as input
  Gain2 : Gain  Gain=sqrt(3)/2  SaturateOnIntegerOverflow=on  OutDataTypeStr=Inherit: Same as input  ParamDataTypeStr=Inherit: Same as input
  Gain3 : Gain  Gain=1/2  SaturateOnIntegerOverflow=on  OutDataTypeStr=Inherit: Same as input  ParamDataTypeStr=Inherit: Same as input
  Gain4 : Gain  Gain=sqrt(3)/2  SaturateOnIntegerOverflow=on  OutDataTypeStr=Inherit: Same as input  ParamDataTypeStr=Inherit: Same as input
  Gain5 : Gain  SaturateOnIntegerOverflow=on  OutDataTypeStr=Inherit: Same as input  ParamDataTypeStr=Inherit: Same as input
  Mux : Mux  Inputs=3
  Sum : Sum  Inputs=-+  SaturateOnIntegerOverflow=on
  Sum1 : Sum  Inputs=--  SaturateOnIntegerOverflow=on
  ABC : Outport
  wires:
  Gain5/1 -> ABC/1
  Mux/1 -> Gain5/1
  Sum1/1 -> Mux/3
  Gain4/1 -> Sum1/2
  Gain3/1 -> Sum1/1
  Sum/1 -> Mux/2
  Gain2/1 -> Sum/2
  Gain1/1 -> Sum/1
  Beta/1 -> Gain4/1, Gain2/1
  Gain/1 -> Mux/1
  Alpha/1 -> Gain1/1, Gain/1, Gain3/1

== system PMSM_FOC_demo/PMSM/iPARK ==
  d : Inport
  q : Inport  Port=2
  theta : Inport  Port=3
  Product{,1..3} (4 alike) : Product  SaturateOnIntegerOverflow=on  OutDataTypeStr=Inherit: Same as first input
  Sum : Sum  Inputs=+-  SaturateOnIntegerOverflow=on
  Sum1 : Sum  SaturateOnIntegerOverflow=on
  Trigonometric Function : Trigonometry
  Trigonometric Function1 : Trigonometry  Operator=cos
  Alpha : Outport
  Beta : Outport  Port=2
  wires:
  Sum/1 -> Alpha/1
  q/1 -> Product3/1, Product1/1
  Trigonometric Function/1 -> Product2/2, Product1/2
  Trigonometric Function1/1 -> Product3/2, Product/2
  d/1 -> Product2/1, Product/1
  theta/1 -> Trigonometric Function1/1, Trigonometric Function/1
  Product/1 -> Sum/1
  Product1/1 -> Sum/2
  Sum1/1 -> Beta/1
  Product2/1 -> Sum1/1
  Product3/1 -> Sum1/2

== system PMSM_FOC_demo/SVPWMCal(TI2812)/INFO ==
  note: Pattern #2:
      | With this pattern, identified as "Hardware-Determined" by Texas Instruments, there is always one PWM channel staying constant for the entire PWM period.
      |  So the number of switching times for this pattern is less than pattern #1. As a result, switching losses will be reduced with Pattern #2.
  note: Pattern #1:
      | With this pattern, identified as "Software-Determined" by Texas Instruments, each PWM channel switches twice per every PWM period.
  note: --------------------------------------------------------------------------------------------------------------------------------------------------------------------
  note: Reference: Application Report SPRA524
      | Space-Vector PWM with TMS320C24x Using H/W & S/W Determined Switching Patterns
      | Zhenyu Yu, Texas Instruments
  note: The objective of the SV PWM technique is to approximate the reference voltage vector (U*) instantaneously
      | by combination of the switching states corresponding to the basic space vectors.
  note: U7 = 1 1 1
  note: Q1 Q3 Q5
  note: --------------------------------------------------------
  note: Three-Phase VSC Diagram
  note: -
  note: +
  note: --------------------------------------------------------
  note: |
      | |
      | |
  note: ---Vc
  note: |
      | |
      | |
  note: |
      | |
      | |
      | |
      | |
      | |
  note: [Q6]
  note: [Q5]
  note: |
      | |
      | |
  note: ---Vb
  note: |
      | |
      | |
  note: |
      | |
      | |
      | |
      | |
      | |
  note: [Q4]
  note: [Q3]
  note: |
      | |
      | |
  note: ---Va
  note: |
      | |
      | |
  note: |
      | |
      | |
      | |
      | |
      | |
  note: [Q2]
  note: [Q1]
  note: Vdc
  note: [n] = Sector number
  note: [2]
  note: Basic Space Vectors and Switching States
  note: U4 = 0 1 1
  note: U5 = 0 0 1
  note: U6 = 1 0 1
  note: U0 = 0 0 0
  note: U3 = 0 1 0
  note: U2 = 1 1 0
  note: U1 = 1 0 0
  note: [6]
  note: [5]
  note: [4]
  note: [3]
  note: [1]
  note: 3                       2
      |       3                   2
      |         3               2
      |           3           2
      |             3       2
      |               3   2
      | 4 4 4 4 4 4 4 4 0 1 1 1 1 1 1 1 1
      |               5   6
      |             5       6
      |           5           6
      |         5               6
      |       5                   6
      |     5                       6
  note: Two symmetrical switching patterns have been implemented:

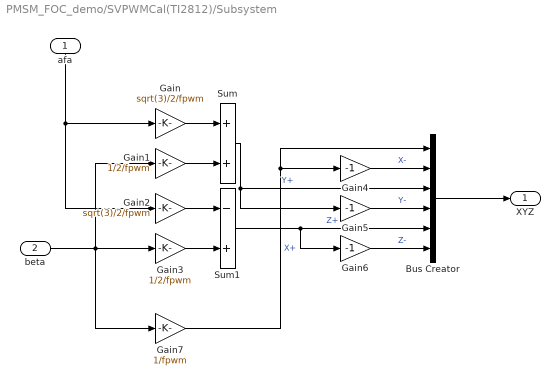
== system PMSM_FOC_demo/SVPWMCal(TI2812)/Subsystem ==
  afa : Inport
  beta : Inport  Port=2
  Bus Creator : BusCreator  Inputs=6
  Gain : Gain  Gain=sqrt(3)/2/fpwm
  Gain1 : Gain  Gain=1/2/fpwm
  Gain2 : Gain  Gain=sqrt(3)/2/fpwm
  Gain3 : Gain  Gain=1/2/fpwm
  Gain4 : Gain  Gain=-1
  Gain5 : Gain  Gain=-1
  Gain6 : Gain  Gain=-1
  Gain7 : Gain  Gain=1/fpwm
  Sum : Sum
  Sum1 : Sum  Inputs=-+
  XYZ : Outport
  wires:
  Gain7/1 -> Bus Creator/1, Gain4/1  "X+"
  Bus Creator/1 -> XYZ/1
  Gain6/1 -> Bus Creator/6  "Z-"
  Sum1/1 -> Bus Creator/5, Gain6/1  "Z+"
  Gain5/1 -> Bus Creator/4  "Y-"
  Sum/1 -> Bus Creator/3, Gain5/1  "Y+"
  Gain4/1 -> Bus Creator/2  "X-"
  beta/1 -> Gain7/1, Gain3/1, Gain1/1
  afa/1 -> Gain2/1, Gain/1
  Gain3/1 -> Sum1/2
  Gain2/1 -> Sum1/1
  Gain1/1 -> Sum/2
  Gain/1 -> Sum/1

== system PMSM_FOC_demo/SVPWMCal(TI2812)/TaTbTcCal ==
  sector : Inport
  ton : Inport  Port=2
  0-60 : Constant  Value=[1 2 3]  VectorParams1D=off  SampleTime=-1
  120-180 : Constant  Value=[3 1 2]  VectorParams1D=off  SampleTime=-1
  180-240 : Constant  Value=[3 2 1]  VectorParams1D=off  SampleTime=-1
  240-300 : Constant  Value=[2 3 1]  VectorParams1D=off  SampleTime=-1
  300-360 : Constant  Value=[1 3 2]  VectorParams1D=off  SampleTime=-1
  60-120 : Constant  Value=[2 1 3]  VectorParams1D=off  SampleTime=-1
  Multiport Switch : MultiPortSwitch  Inputs=6
  Selector : Selector  InputPortWidth=3  IndexOptions=Index vector (port)  Indices=[1 3]  OutputSizes=1
  TaTbTc : Outport
  wires:
  Selector/1 -> TaTbTc/1
  ton/1 -> Selector/1
  sector/1 -> Multiport Switch/1
  Multiport Switch/1 -> Selector/2
  300-360/1 -> Multiport Switch/7
  240-300/1 -> Multiport Switch/6
  180-240/1 -> Multiport Switch/5
  120-180/1 -> Multiport Switch/4
  60-120/1 -> Multiport Switch/3
  0-60/1 -> Multiport Switch/2

== system PMSM_FOC_demo/SVPWMCal(TI2812)/sector ==
  afa : Inport
  beta : Inport  Port=2
  Cartesian to Polar : simulink_extras/Transformations/Cartesian to Polar
  Constant2 : Constant  Value=2*pi  SampleTime=ts_cc
  Look-Up Table : Lookup  InputValues=[0:pi/3:5*pi/3]  Table=[1:6]  SaturateOnIntegerOverflow=on
  Math Function2 : Math  Operator=mod  SaturateOnIntegerOverflow=on
  Rounding Function : Rounding
  Saturation : Saturate  UpperLimit=6  LowerLimit=1
  Terminator : Terminator
  sector : Outport
  wires:
  Saturation/1 -> Rounding Function/1
  Rounding Function/1 -> sector/1
  beta/1 -> Cartesian to Polar/2
  afa/1 -> Cartesian to Polar/1
  Cartesian to Polar/2 -> Math Function2/1
  Math Function2/1 -> Look-Up Table/1
  Constant2/1 -> Math Function2/2
  Look-Up Table/1 -> Saturation/1
  Cartesian to Polar/1 -> Terminator/1

== system PMSM_FOC_demo/SVPWMCal(TI2812)/t1 t2 ==
  sector : Inport
  XYZ : Inport  Port=2
  0-60 : Constant  Value=[6 1]  VectorParams1D=off  SampleTime=-1
  120-180 : Constant  Value=[1 4]  VectorParams1D=off  SampleTime=-1
  180-240 : Constant  Value=[2 5]  VectorParams1D=off  SampleTime=-1
  240-300 : Constant  Value=[4 6]  VectorParams1D=off  SampleTime=-1
  300-360 : Constant  Value=[3 2]  VectorParams1D=off  SampleTime=-1
  60-120 : Constant  Value=[5 3]  VectorParams1D=off  SampleTime=-1
  Multiport Switch : MultiPortSwitch  Inputs=6
  Selector : Selector  InputPortWidth=6  IndexOptions=Index vector (port)  Indices=[1 3]  OutputSizes=1
  t1 t2 : Outport
  wires:
  Selector/1 -> t1 t2/1
  XYZ/1 -> Selector/1
  sector/1 -> Multiport Switch/1
  Multiport Switch/1 -> Selector/2
  300-360/1 -> Multiport Switch/7
  240-300/1 -> Multiport Switch/6
  180-240/1 -> Multiport Switch/5
  120-180/1 -> Multiport Switch/4
  60-120/1 -> Multiport Switch/3
  0-60/1 -> Multiport Switch/2

== system PMSM_FOC_demo/SVPWMCal(TI2812)/ton ==
  t1 t2 : Inport
  Bus Creator : BusCreator  Inputs=3
  Demux : Demux  Outputs=2
  Fcn : Fcn  Expr=(1/fpwm-u(1)-u(2))/2
  Sum : Sum  Inputs=|++
  Sum1 : Sum  Inputs=++|
  ton : Outport
  wires:
  Bus Creator/1 -> ton/1
  Sum1/1 -> Bus Creator/3  "tcon"
  Sum/1 -> Sum1/1, Bus Creator/2  "tbon"
  Demux/2 -> Sum1/2
  Demux/1 -> Sum/2
  Fcn/1 -> Bus Creator/1, Sum/1  "taon"
  t1 t2/1 -> Fcn/1, Demux/1

== system PMSM_FOC_demo/Sensors&SignalConditioning/DcLinkVolt ==
  In1 : Inport
  Constant : Constant  Value=Offset
  Gain : Gain  Gain=Gain
  Sum : Sum  Inputs=|++
  Out1 : Outport
  wires:
  Gain/1 -> Sum/1
  Constant/1 -> Sum/2
  In1/1 -> Gain/1
  Sum/1 -> Out1/1

== system PMSM_FOC_demo/Sensors&SignalConditioning/PhACurrConditioning ==
  In1 : Inport
  Constant : Constant  Value=Offset
  Gain : Gain  Gain=Gain
  Sum : Sum  Inputs=|++
  Out1 : Outport
  wires:
  In1/1 -> Gain/1
  Constant/1 -> Sum/2
  Gain/1 -> Sum/1
  Sum/1 -> Out1/1

== system PMSM_FOC_demo/Sensors&SignalConditioning/PhACurrConditioning1 ==
  In1 : Inport
  Constant : Constant  Value=Offset
  Gain : Gain  Gain=Gain
  Sum : Sum  Inputs=|++
  Out1 : Outport
  wires:
  Sum/1 -> Out1/1
  Gain/1 -> Sum/1
  Constant/1 -> Sum/2
  In1/1 -> Gain/1

== system PMSM_FOC_demo/Sensors&SignalConditioning/ResolverConditioning ==
  pos : Inport
  spd : Inport  Port=2
  theta_m : Outport
  omega_m : Outport  Port=2
  wires:
  spd/1 -> omega_m/1
  pos/1 -> theta_m/1

== system PMSM_FOC_demo/Controller/CurrentParkTrans/CLARK (32) ==
  ABC : Inport
  Demux : Demux  Outputs=3
  Gain : Gain  SaturateOnIntegerOverflow=on  OutDataTypeStr=Inherit: Same as input  ParamDataTypeStr=Inherit: Same as input
  Gain1 : Gain  Gain=1/2  SaturateOnIntegerOverflow=on  OutDataTypeStr=Inherit: Same as input  ParamDataTypeStr=Inherit: Same as input
  Gain2 : Gain  Gain=1/2  SaturateOnIntegerOverflow=on  OutDataTypeStr=Inherit: Same as input  ParamDataTypeStr=Inherit: Same as input
  Gain3 : Gain  Gain=sqrt(3)/2  SaturateOnIntegerOverflow=on  OutDataTypeStr=Inherit: Same as input  ParamDataTypeStr=Inherit: Same as input
  Gain4 : Gain  Gain=sqrt(3)/2  SaturateOnIntegerOverflow=on  OutDataTypeStr=Inherit: Same as input  ParamDataTypeStr=Inherit: Same as input
  Gain5 : Gain  Gain=2/3  SaturateOnIntegerOverflow=on  OutDataTypeStr=Inherit: Same as input  ParamDataTypeStr=Inherit: Same as input
  Mux : Mux  Inputs=2
  Sum : Sum  Inputs=+--  SaturateOnIntegerOverflow=on
  Sum1 : Sum  Inputs=+-  SaturateOnIntegerOverflow=on
  AlphaBeta : Outport
  wires:
  Gain4/1 -> Sum1/2
  Gain3/1 -> Sum1/1
  Gain2/1 -> Sum/3
  Gain1/1 -> Sum/2
  Gain/1 -> Sum/1
  Demux/3 -> Gain4/1, Gain2/1
  Demux/2 -> Gain3/1, Gain1/1
  Demux/1 -> Gain/1
  ABC/1 -> Gain5/1
  Mux/1 -> AlphaBeta/1
  Sum/1 -> Mux/1
  Sum1/1 -> Mux/2
  Gain5/1 -> Demux/1

== system PMSM_FOC_demo/Controller/CurrentParkTrans/PARK ==
  AlphaBeta : Inport
  Theta : Inport  Port=2
  Demux : Demux  Outputs=2
  Mux : Mux  Inputs=2
  Product{,1..3} (4 alike) : Product  SaturateOnIntegerOverflow=on  OutDataTypeStr=Inherit: Same as first input
  Sum : Sum  SaturateOnIntegerOverflow=on
  Sum1 : Sum  Inputs=-+  SaturateOnIntegerOverflow=on
  Trigonometric Function : Trigonometry  Operator=cos
  Trigonometric Function1 : Trigonometry
  dq : Outport
  wires:
  Product2/1 -> Sum1/1
  Theta/1 -> Trigonometric Function/1, Trigonometric Function1/1
  Trigonometric Function/1 -> Product/2, Product3/1
  Product/1 -> Sum/1
  Trigonometric Function1/1 -> Product1/2, Product2/2
  Demux/2 -> Product1/1, Product3/2
  Product1/1 -> Sum/2
  Product3/1 -> Sum1/2
  Demux/1 -> Product/1, Product2/1
  AlphaBeta/1 -> Demux/1
  Mux/1 -> dq/1
  Sum/1 -> Mux/1
  Sum1/1 -> Mux/2

== system PMSM_FOC_demo/PMSM/ElectricalMod/dAxisVolEqu ==
  Ud : Inport
  w : Inport  Port=2
  iq : Inport  Port=3
  Gain1 : Gain  Gain=Lq  SaturateOnIntegerOverflow=on  OutDataTypeStr=Inherit: Same as input  ParamDataTypeStr=Inherit: Same as input
  Product : Product  SaturateOnIntegerOverflow=on  OutDataTypeStr=Inherit: Same as first input
  Scope1 : Scope  NumInputPorts=2
  Scope2 : Scope  NumInputPorts=2
  Sum : Sum  SaturateOnIntegerOverflow=on
  Transfer Fcn : TransferFcn  Denominator=[Ld r]
  lamdaq : Outport
  id : Outport  Port=2
  wires:
  Ud/1 -> Sum/1
  Transfer Fcn/1 -> id/1, Scope1/1
  Sum/1 -> Transfer Fcn/1, Scope1/2
  Product/1 -> Scope2/1, Sum/2
  w/1 -> Product/1
  Gain1/1 -> Product/2, lamdaq/1
  iq/1 -> Scope2/2, Gain1/1

== system PMSM_FOC_demo/PMSM/ElectricalMod/qAxisVolEqu ==
  id : Inport
  w : Inport  Port=2
  Uq : Inport  Port=3
  Add : Sum
  Constant : Constant  Value=lamdaPM
  Gain1 : Gain  Gain=Ld  SaturateOnIntegerOverflow=on  OutDataTypeStr=Inherit: Same as input  ParamDataTypeStr=Inherit: Same as input
  Product : Product  SaturateOnIntegerOverflow=on  OutDataTypeStr=Inherit: Same as first input
  Scope3 : Scope  NumInputPorts=3
  Sum : Sum  Inputs=+-  SaturateOnIntegerOverflow=on
  Transfer Fcn : TransferFcn  Denominator=[Lq r]
  iq : Outport
  lamdad : Outport  Port=2
  wires:
  Constant/1 -> Add/2
  Add/1 -> lamdad/1, Product/2
  Gain1/1 -> Add/1
  Transfer Fcn/1 -> Scope3/1, iq/1
  Sum/1 -> Transfer Fcn/1
  Product/1 -> Scope3/3, Sum/2
  w/1 -> Product/1
  id/1 -> Gain1/1
  Uq/1 -> Scope3/2, Sum/1
